simulink model "matprod"  (R2015a)
settings: Solver=ode45  StartTime=0.0  StopTime=10.0  RelTol=1e-3
settings Model: Creator=shohei  LastModifiedBy=shohei

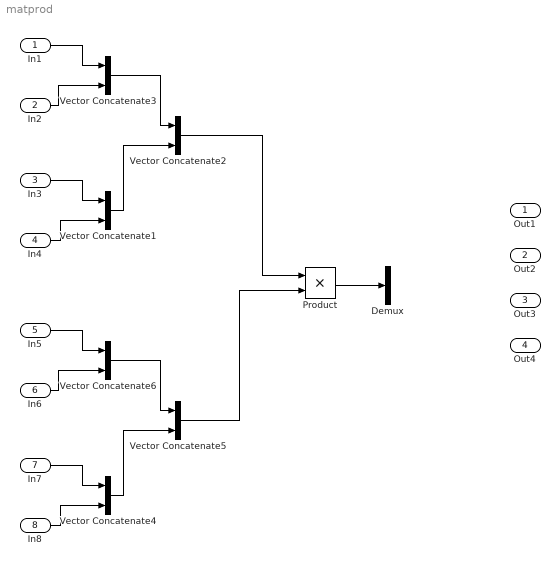
== system matprod ==
  In1 : Inport
  In2 : Inport  Port=2
  In3 : Inport  Port=3
  In4 : Inport  Port=4
  In5 : Inport  Port=5
  In6 : Inport  Port=6
  In7 : Inport  Port=7
  In8 : Inport  Port=8
  Demux : Demux  Outputs=2
  Product : Product
  Vector Concatenate{1,3..4,6} (4 alike) : Concatenate  Mode=Multidimensional array  ConcatenateDimension=2
  Vector Concatenate2 : Concatenate  Mode=Multidimensional array
  Vector Concatenate5 : Concatenate  Mode=Multidimensional array
  Out1 : Outport
  Out2 : Outport  Port=2
  Out3 : Outport  Port=3
  Out4 : Outport  Port=4
  wires:
  In3/1 -> Vector Concatenate1/1
  In4/1 -> Vector Concatenate1/2
  Vector Concatenate1/1 -> Vector Concatenate2/2
  In1/1 -> Vector Concatenate3/1
  In2/1 -> Vector Concatenate3/2
  Vector Concatenate3/1 -> Vector Concatenate2/1
  In7/1 -> Vector Concatenate4/1
  In8/1 -> Vector Concatenate4/2
  Vector Concatenate4/1 -> Vector Concatenate5/2
  In5/1 -> Vector Concatenate6/1
  In6/1 -> Vector Concatenate6/2
  Vector Concatenate6/1 -> Vector Concatenate5/1
  Vector Concatenate2/1 -> Product/1
  Vector Concatenate5/1 -> Product/2
  Product/1 -> Demux/1
